simulink model "Linear_Plant"  (R2024b)
settings: Solver=VariableStepAuto  StartTime=0.0  StopTime=300  RelTol=1e-3
settings Model: Creator=aryaman  LastModifiedBy=aryaman
settings DataIOCC: SaveFormat=StructureWithTime

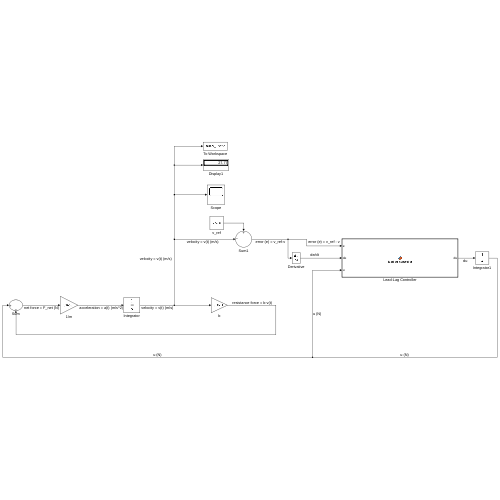
[thumbnail: Simulink's stored preview of the top-level diagram]
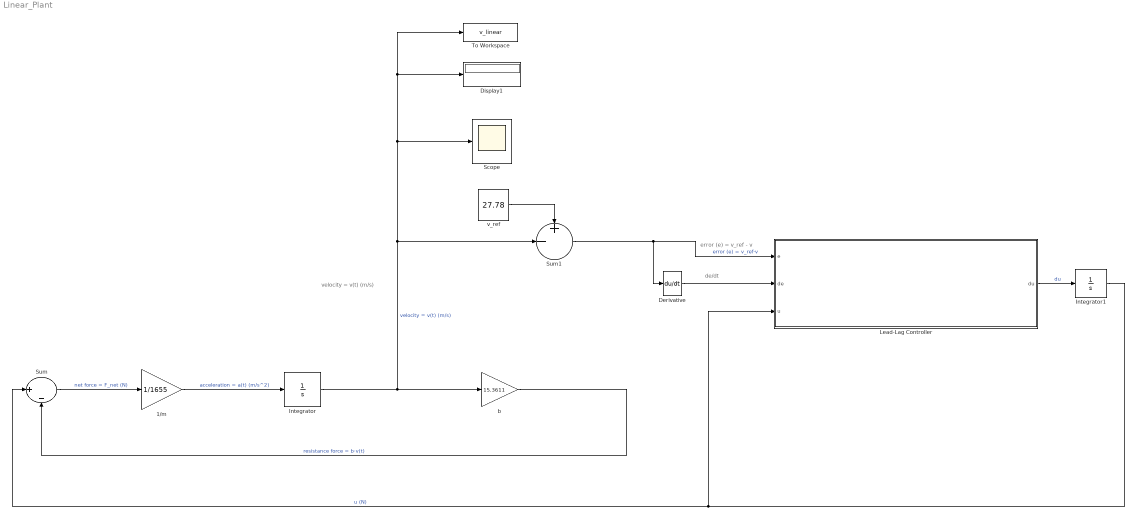
== system Linear_Plant ==
  note: de/dt
  note: error (e) = v_ref - v
  note: velocity = v(t) (m/s)
  1/m : Gain  Gain=1/1655
  Derivative : Derivative
  Display1 : Display
  Integrator : Integrator
  Integrator1 : Integrator
  Lead-Lag Controller : MATLAB Function  TreatAsAtomicUnit=on
  Scope : Scope
  Sum : Sum  Inputs=||+|-
  Sum1 : Sum  Inputs=+-|
  To Workspace : ToWorkspace  VariableName=v_linear  SampleTime=-1
  b : Gain  Gain=15.3611
  v_ref : Constant  Value=27.78
  wires:
  Sum/1 -> 1/m/1  "net force = F_net (N)"
  1/m/1 -> Integrator/1  "acceleration = a(t) (m/s^2)"
  Integrator/1 -> b/1, Display1/1, To Workspace/1, Scope/1, Sum1/2  "velocity = v(t) (m/s)"
  b/1 -> Sum/2  "resistance force = b·v(t)"
  v_ref/1 -> Sum1/1
  Sum1/1 -> Derivative/1, Lead-Lag Controller/1(e)  "error (e) = v_ref-v"
  Derivative/1 -> Lead-Lag Controller/2(de)
  Lead-Lag Controller/1(du) -> Integrator1/1  "du"
  Integrator1/1 -> Lead-Lag Controller/3(u), Sum/1  "u (N)"

== matlab function Linear_Plant/Lead-Lag Controller ==
  data: e input; du output; de input; u input
function du = leadlag_controller(e, de, u)
% e = error = v_ref - v

% Controller parameters
K = 50;
z = 2.40;
p = 0.050;

% Lead-Lag Transfer Function
% C(s) = U(s)/E(s)
%C = K * (s + z) / (s + p);

du = K*(de + z*e) - p*u;

end
